simulink model "nonlinear_without_noise"  (R2020a)
settings: Solver=VariableStepAuto  StartTime=0.0  StopTime=10  RelTol=1e-3
settings Model: Creator=Navid  LastModifiedBy=emami

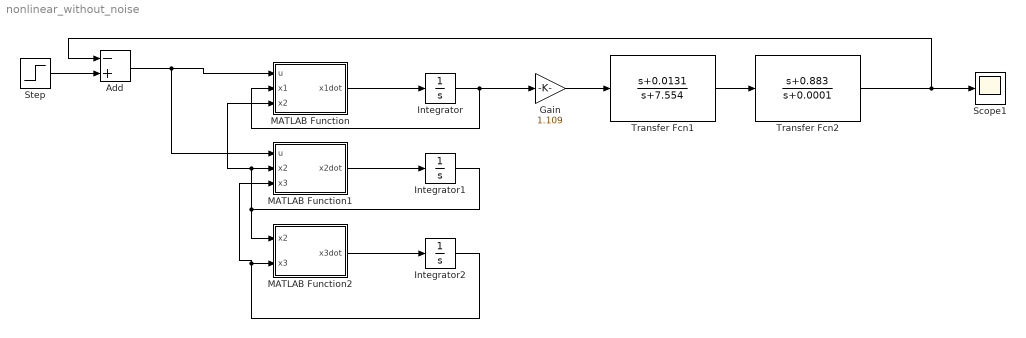
== system nonlinear_without_noise ==
  Add : Sum  Inputs=-+
  Gain : Gain  Gain=1.109
  Integrator : Integrator  InitialCondition=0.00001  IgnoreLimit=on
  Integrator1 : Integrator  InitialCondition=0.00001
  Integrator2 : Integrator  InitialCondition=0.00001
  MATLAB Function : MATLAB Function  TreatAsAtomicUnit=on
  MATLAB Function1 : MATLAB Function  TreatAsAtomicUnit=on
  MATLAB Function2 : MATLAB Function  TreatAsAtomicUnit=on
  Scope1 : Scope
  Step : Step  SampleTime=0
  Transfer Fcn1 : TransferFcn  Numerator=[1 0.0131]  Denominator=[1 7.554]
  Transfer Fcn2 : TransferFcn  Numerator=[1 0.883]  Denominator=[1 0.0001]
  wires:
  Gain/1 -> Transfer Fcn1/1
  MATLAB Function/1(x1dot) -> Integrator/1
  MATLAB Function2/1(x3dot) -> Integrator2/1
  Transfer Fcn1/1 -> Transfer Fcn2/1
  Integrator1/1 -> MATLAB Function/3(x2), MATLAB Function1/2(x2), MATLAB Function2/1(x2)
  Integrator2/1 -> MATLAB Function1/3(x3), MATLAB Function2/2(x3)
  MATLAB Function1/1(x2dot) -> Integrator1/1
  Integrator/1 -> Gain/1, MATLAB Function/2(x1)
  Step/1 -> Add/2
  Add/1 -> MATLAB Function1/1(u), MATLAB Function/1(u)
  Transfer Fcn2/1 -> Scope1/1, Add/1

== matlab function nonlinear_without_noise/MATLAB Function ==
  data: u input; x1dot output; x1 input; x2 input
function x1dot = fcn(u,x1,x2)
u5 = 3270.*(360*u+1.4-x1.*(u+0.005))./x2;
x1dot = u5;

== matlab function nonlinear_without_noise/MATLAB Function2 ==
  data: x3dot output; x2 input; x3 input
function x3dot = fcn(x2,x3)
x3dot = 10010*((x2-x3)/10^5 - x3/(1.5*10^5));

== matlab function nonlinear_without_noise/MATLAB Function1 ==
  data: u input; x2dot output; x2 input; x3 input
function x2dot = fcn(u,x2,x3)
x2dot = 3270*(u+0.005-(x2-x3)/10^5);
